simulink model "PlantaV4_6_prueba_contacto_4"  (R2021a)
settings: Solver=VariableStepAuto  StartTime=0.0  StopTime=60  MaxStep=1e-2  RelTol=1e-3
values from neighbouring files (symbols this model uses):
  ahmax = 0.75    [valoresPlanta_29_9_24.m]    (also in valoresPlanta_V3.m)
  alfahmax = ((2*ahmax)/(rhd))    (= 2)    [valoresPlanta_29_9_24.m]    (also in valoresPlanta_V3.m)
  alfatmax = atmax/rtd    (= 1.6)    [valoresPlanta_29_9_24.m]    (also in valoresPlanta_V3.m)
  atmax = 0.8    [valoresPlanta_29_9_24.m]    (also in valoresPlanta_V3.m)
  ax_max = 0.8    [valoresPlanta_29_9_24.m]    (also in valoresPlanta_v4.m)
  ay_max = 0.75    [valoresPlanta_29_9_24.m]    (also in valoresPlanta_v4.m)
  bcx = 1e6    (= 1000000)    [Valores_1.m]    (also in valoresPlanta.m; valoresPlanta_29_9_24.m; valoresPlanta_V3.m; valoresPlanta_v4.m)
  bcy = 1e7    (= 10000000)    [Valores_1.m]    (also in valoresPlanta.m; valoresPlanta_29_9_24.m; valoresPlanta_V3.m; valoresPlanta_v4.m)
  bh_eq = bhm*ih^2+bhd    (= 8720)    [Valores.m]    (also in Valores_1.m; valoresPlanta.m; valoresPlanta_29_9_24.m; valoresPlanta_V3.m)
  bhb = 1e8    (= 100000000)    [Valores.m]    (also in Valores_1.m; valoresPlanta.m; valoresPlanta_29_9_24.m; valoresPlanta_V3.m)
  bhEb = 2.2e9    (= 2200000000)    [Valores.m]    (also in Valores_1.m; valoresPlanta.m; valoresPlanta_29_9_24.m; valoresPlanta_V3.m)
  bt = 90.0    (= 90)    [Valores.m]    (also in Valores_1.m; valoresPlanta.m; valoresPlanta_29_9_24.m; valoresPlanta_V3.m)
  bt_eq = btd+(btm*(it^2))    (= 5401.8)    [valoresPlanta.m]    (also in valoresPlanta_29_9_24.m; valoresPlanta_V3.m; valoresPlanta_v4.m)
  btw = 3.0e3    (= 3000)    [Valores.m]    (also in Valores_1.m; valoresPlanta.m; valoresPlanta_29_9_24.m; valoresPlanta_V3.m)
  bwu = 150    [Valores.m]    (also in Valores_1.m; valoresPlanta.m; valoresPlanta_29_9_24.m; valoresPlanta_V3.m)
  estado_cont = [x_positions; hy_cont]    [perfilObsaculos.m]    (also in valoresPlanta_29_9_24.m = [x_positions; [hy_muelle hy_cont]])
  g = 9.80665    [Valores.m]    (also in Valores_1.m; valoresPlanta.m; valoresPlanta_29_9_24.m; valoresPlanta_V3.m)
  Hc = 0    [Valores.m]    (also in Valores_1.m = 2.5; valoresPlanta.m = 2.5; valoresPlanta_29_9_24.m = 2.5; valoresPlanta_V3.m = 2.5)
  hMax = 10    [Valores_1.m]    (also in valoresPlanta.m; valoresPlanta_V3.m; valoresPlanta_v4.m)
  hx_cont = 2.5    [perfilObsaculos.m]    (also in puntosTrayectoria.m; valoresPlanta_29_9_24.m)
  ih = 22    [Valores.m]    (also in Valores_1.m; valoresPlanta.m; valoresPlanta_29_9_24.m; valoresPlanta_V3.m)
  it = 30    [Valores.m]    (also in Valores_1.m; valoresPlanta.m; valoresPlanta_29_9_24.m; valoresPlanta_V3.m)
  Jh_eq = Jhm_hb*ih^2+Jhd_hEb    (= 18320)    [Valores.m]    (also in Valores_1.m; valoresPlanta.m; valoresPlanta_29_9_24.m; valoresPlanta_V3.m)
  Jt_eq = Jtd+(Jtm_tb*(it^2))    (= 7500)    [valoresPlanta.m]    (also in valoresPlanta_29_9_24.m; valoresPlanta_V3.m; valoresPlanta_v4.m)
  kcy = 1.8e9    (= 1800000000)    [Valores_1.m]    (also in valoresPlanta.m; valoresPlanta_29_9_24.m; valoresPlanta_V3.m; valoresPlanta_v4.m)
  KDh = Jeq2 * w_posh^3    (= -12245.4404091)    [Valores.m]    (also in Valores_1.m = Jeq2 * w_posh; valoresPlanta.m = Jeq2 * w_posh; valoresPlanta_29_9_24.m = Jh_eq * n * w_posh; valoresPlanta_V3.m = Jeq2 * w_posh)
  KDt = Meq2 * w_post^3    (= -4728.86946035)    [Valores.m]    (also in Valores_1.m = Meq2 * w_post; valoresPlanta.m = Meq2 * w_post; valoresPlanta_29_9_24.m = 10127; valoresPlanta_V3.m = Meq2 * w_post)
  KIh = Jeq2 * w_posh^2    (= 2572.66592082)    [Valores.m]    (also in Valores_1.m = Jeq2 * w_posh^3; valoresPlanta.m = Jeq2 * w_posh^3; valoresPlanta_29_9_24.m = Jh_eq * w_posh^3; valoresPlanta_V3.m = Jeq2 * w_posh^3)
  KIt = Meq2 * w_post^2    (= 1307.690244)    [Valores.m]    (also in Valores_1.m = Meq2 * w_post^3; valoresPlanta.m = Meq2 * w_post^3; valoresPlanta_29_9_24.m = 6809.6; valoresPlanta_V3.m = Meq2 * w_post^3)
  KPh = Jeq2 * w_posh    (= -540.495867769)    [Valores.m]    (also in Valores_1.m = Jeq2 * w_posh^2; valoresPlanta.m = Jeq2 * w_posh^2; valoresPlanta_29_9_24.m = Jh_eq * n * w_posh^2; valoresPlanta_V3.m = Jeq2 * w_posh^2)
  KPt = Meq2 * w_post    (= -361.62)    [Valores.m]    (also in Valores_1.m = Meq2 * w_post^2; valoresPlanta.m = Meq2 * w_post^2; valoresPlanta_29_9_24.m = 14123; valoresPlanta_V3.m = Meq2 * w_post^2)
  Ktw = 4.8e5    (= 480000)    [Valores.m]    (also in Valores_1.m; valoresPlanta.m; valoresPlanta_29_9_24.m; valoresPlanta_V3.m)
  kwu = 2.36e8    (= 236000000)    [Valores.m]    (also in Valores_1.m; valoresPlanta.m; valoresPlanta_29_9_24.m; valoresPlanta_V3.m)
  Mc_max = 5e4    (= 50000)    [Valores.m]    (also in Valores_1.m; valoresPlanta.m; valoresPlanta_29_9_24.m; valoresPlanta_V3.m)
  Mc_min = 2e3    (= 2000)    [Valores.m]    (also in Valores_1.m; valoresPlanta.m; valoresPlanta_29_9_24.m; valoresPlanta_V3.m)
  Meq = Mt+(it^2*Jtm_tb+Jtd)/rtd^2    (= 60000)    [Valores.m]    (also in Valores_1.m; valoresPlanta_29_9_24.m; valoresPlanta_v4.m)
  Ms = 1.5e4    (= 15000)    [Valores.m]    (also in Valores_1.m; valoresPlanta.m; valoresPlanta_29_9_24.m; valoresPlanta_V3.m)
  Mt = 30000    [Valores.m]    (also in Valores_1.m; valoresPlanta.m; valoresPlanta_29_9_24.m; valoresPlanta_V3.m)
  rhd = 0.75    [Valores.m]    (also in Valores_1.m; valoresPlanta.m; valoresPlanta_29_9_24.m; valoresPlanta_V3.m)
  rtd = 0.5    [Valores.m]    (also in Valores_1.m; valoresPlanta.m; valoresPlanta_29_9_24.m; valoresPlanta_V3.m)
  tau_hm = 1e-3    (= 0.001)    [valoresPlanta.m]    (also in valoresPlanta_29_9_24.m; valoresPlanta_V3.m; valoresPlanta_v4.m)
  tau_tm = 1e-3    (= 0.001)    [Valores.m]    (also in Valores_1.m; valoresPlanta.m; valoresPlanta_29_9_24.m; valoresPlanta_V3.m)
  Thb_Max = 5e4    (= 50000)    [Valores.m]    (also in Valores_1.m; valoresPlanta.m; valoresPlanta_29_9_24.m; valoresPlanta_V3.m)
  ThEb_Max = 1.1e6    (= 1100000)    [Valores.m]    (also in Valores_1.m; valoresPlanta.m; valoresPlanta_29_9_24.m; valoresPlanta_V3.m)
  Thm_Max = 2e4    (= 20000)    [Valores.m]    (also in Valores_1.m; valoresPlanta.m; valoresPlanta_29_9_24.m; valoresPlanta_V3.m)
  Ttb_Max = 5e3    (= 5000)    [Valores.m]    (also in Valores_1.m; valoresPlanta.m; valoresPlanta_29_9_24.m; valoresPlanta_V3.m)
  Ttm_Max = 3e3    (= 3000)    [Valores.m]    (also in Valores_1.m; valoresPlanta.m; valoresPlanta_29_9_24.m = 4000; valoresPlanta_V3.m)
  v_x_max = 4    [Valores_1.m]    (also in valoresPlanta.m; valoresPlanta_V3.m = 0.4; valoresPlanta_v4.m)
  vx_max = 4    [valoresPlanta_29_9_24.m]
  y0 = 2.5    [valoresPlanta_29_9_24.m]
  Yt0 = 45    [Valores.m]    (also in Valores_1.m; valoresPlanta.m; valoresPlanta_29_9_24.m; valoresPlanta_V3.m)
undefined symbols (not defined in the file or in its folder): sigbuilder_block, x0
libraries: vrlib x1, simulink_extras x1, cstblocks x1
(part 1 of 2)
settings Model: Creator=Matias  LastModifiedBy=agustin

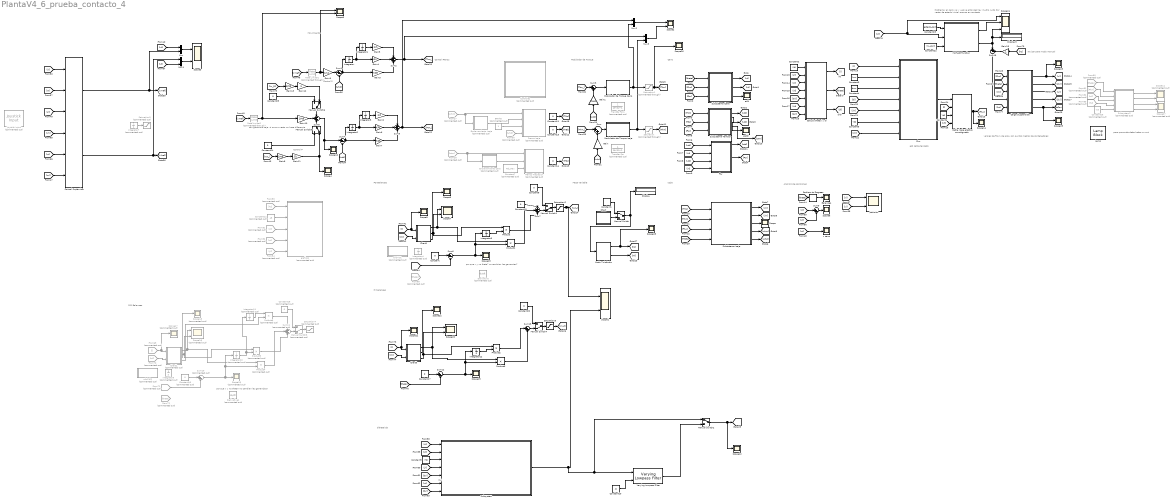
== system PlantaV4_6_prueba_contacto_4 ==
  note: para que ande debe haber un out
  note: revisar para modo manual
  note: ec2 cable tensado
  note: Problema: el carro va y vuelve entonces hay mucho ruido
      | Por vector de estado inicial arranco en contacto
  note: PI balanceo
  note: con ganancia baja, si sumo o resto no hace diferencia
  note: Control P
  note: por que v y no theta? no cambian las ganancias?
  note: d(theta)/dt
  note: Analisis de posiciones
  note: PD Balanceo
  note: Masa Variable
  note: Control Frenos
  note: Izaje
  note: Modulador de Torque
  note: Carro
  note: Movimiento
  note: PID Balanceo
  note: por que v y no theta? no cambian las ganancias?
  note: Control P
  note: valores de fila 1 de array son puntos medios de contenedores
  In4 : Inport
  BRKhE : Constant  Commented=on
  Balanceo : Scope
  Cable izaje elástico amortiguado : Subsystem
  Calculo theta,l y dl : Subsystem
  Carga Suspendida : Subsystem
  Chart : Stateflow chart  TreatAsAtomicUnit=on
  Chart1 : Stateflow chart  TreatAsAtomicUnit=on
  Chart2 : Stateflow chart  Commented=on  TreatAsAtomicUnit=on
  Chart3 : Stateflow chart  TreatAsAtomicUnit=on
  Constant{,8,11,13..15,17,20,24..25} (10 alike) : Constant  Value=0
  Constant1 : Constant  Value=65000
  Constant10 : Constant  Value=.8
  Constant12 : Constant  Commented=on  Value=45
  Constant16 : Constant  Commented=on  Value=0
  Constant18 : Constant  Commented=on  Value=0
  Constant{2,5..6,9} (4 alike) : Constant  Value=Yt0
  Constant22 : Constant  Value=hx_cont
  Constant23 : Constant  Value=estado_cont
  Constant26 : Constant  Commented=on  Value=-10
  Constant3 : Constant  Value=kwu
  Constant4 : Constant  Value=bwu
  Constant7 : Constant  Commented=on  Value=Ttb_Max
  Control Supervisor : Subsystem
  Controles : Subsystem  Commented=on
  Derivative : Derivative  Commented=on
  Derivative1 : Derivative  Commented=on
  Display : Display
  Display3 : Display
  Enclavamiento carro : Stateflow chart  Commented=on  TreatAsAtomicUnit=on
  Enclavamiento izaje : Stateflow chart  Commented=on  TreatAsAtomicUnit=on
  Fhw : Subsystem
  "Frenos Izaje " : Stateflow chart  Commented=on  TreatAsAtomicUnit=on
  Frenos Traslación : Stateflow chart  Commented=on  TreatAsAtomicUnit=on
  From27 : From  Commented=on  GotoTag=whm
  From28 : From  Commented=on  GotoTag=wtm
  From30 : From  Commented=on  GotoTag=whd
  From51 : From  Commented=on  GotoTag=xl
  From52 : From  Commented=on  GotoTag=xt
  From53 : From  Commented=on  GotoTag=hc
  From54 : From  Commented=on  GotoTag=yl
  From68 : From  Commented=on  GotoTag=theta
  From69 : From  Commented=on  GotoTag=l
  From70 : From  Commented=on  GotoTag=ml
  From71 : From  Commented=on  GotoTag=dTheta
  From72 : From  Commented=on  GotoTag=theta
  From80 : From  Commented=on  GotoTag=theta
  From81 : From  Commented=on  GotoTag=Fhw
  From82 : From  Commented=on  GotoTag=ml
  From83 : From  Commented=on  GotoTag=hc
  Ftw : Subsystem
  Gain : Gain  Gain=bh_eq
  Gain1 : Gain  Gain=bt_eq
  Gain10 : Gain  Gain=1/rtd
  Gain11 : Gain  Gain=.01
  Gain12 : Gain  Gain=.1
  Gain13 : Gain  Gain=1/rtd
  Gain15 : Gain
  Gain2 : Gain  Gain=KIt
  Gain3 : Gain  Gain=KDh
  Gain4 : Gain  Gain=KPh
  Gain5 : Gain  Gain=KIh
  Gain6 : Gain  Gain=KPt
  Gain7 : Gain  Gain=KDt
  Gain8 : Gain  Gain=1/rtd
  Gain9 : Gain  Gain=2/rhd
  Integrator{,1..3,5,12} (6 alike) : Integrator
  Integrator{4,7,9..11} (5 alike) : Integrator  Commented=on
  Joystick Input : vrlib/Joystick Input  Commented=on  joyid=1  adjustports=on  forcefeed=off
  Lamp : LampBlock
  MATLAB Function : MATLAB Function  TreatAsAtomicUnit=on
  Manual Switch : ManualSwitch
  Manual Switch{1,4..6} (4 alike) : ManualSwitch  CurrentSetting=0
  Manual Switch2 : ManualSwitch
  Manual Switch3 : ManualSwitch  Commented=on  CurrentSetting=0
  Modo Twistlocks : Stateflow chart  TreatAsAtomicUnit=on
  Modulador de Torque Carro : Subsystem
  Modulador de Torque Izaje : Subsystem
  Mux{,1..3} (4 alike) : Mux  Inputs=2
  Product{,1..2,6} (4 alike) : Product
  Product3 : Product  Commented=on
  Product4 : Product  Commented=on
  Product5 : Product  Commented=on
  Radians to Degrees : simulink_extras/Transformations/Radians to Degrees
  Rate Limiter1 : RateLimiter  Commented=through  RisingSlewLimit=ay_max  FallingSlewLimit=-ay_max  SampleTimeMode=inherited
  Rate Limiter2 : RateLimiter  Commented=through  RisingSlewLimit=ax_max  FallingSlewLimit=-ax_max  SampleTimeMode=inherited
  Saturation : Saturate  Commented=through  UpperLimit=Thm_Max  LowerLimit=-Thm_Max
  Saturation1 : Saturate  Commented=through  UpperLimit=Ttm_Max  LowerLimit=-Ttm_Max
  Saturation2 : Saturate  UpperLimit=4  LowerLimit=-4
  Saturation3 : Saturate  Commented=on  UpperLimit=v_x_max  LowerLimit=-4
  Saturation4 : Saturate  Commented=on  UpperLimit=4  LowerLimit=-4
  Saturation5 : Saturate  UpperLimit=4  LowerLimit=-4
  Scope{,4,6,8..10,12..14,19,21..23,25..26,28} (16 alike) : Scope
  Scope{1..3,5,7,20} (6 alike) : Scope  NumInputPorts=2
  Scope11 : Scope  Commented=on  NumInputPorts=2
  Scope15 : Scope  Commented=on
  Scope16 : Scope  Commented=on  NumInputPorts=2
  Scope17 : Scope  Commented=on
  Scope18 : Scope  Commented=on
  Scope24 : Scope  NumInputPorts=3
  Scope27 : Scope  Commented=on  NumInputPorts=2
  Subsistema Carro : Subsystem
  Subsistema Izaje : Subsystem
  Subsistema Tambor : Subsystem
  Subsystem : Subsystem
  Subsystem2 : Subsystem  Commented=on
  Sum : Sum  Inputs=|++
  Sum{1,4,6,9,12,15} (6 alike) : Sum  Inputs=|+-
  Sum10 : Sum  Commented=on  Inputs=|+-
  Sum11 : Sum  Commented=on  Inputs=+++
  Sum13 : Sum  Inputs=|++
  Sum2 : Sum  Inputs=+++
  Sum3 : Sum  Inputs=|++
  Sum5 : Sum  Inputs=+++
  Sum7 : Sum  Inputs=+++
  Sum8 : Sum  Inputs=-++
  Transfer Fcn : TransferFcn  Commented=on  Denominator=[1e-3 1]
  Transfer Fcn1 : TransferFcn  Commented=on  Denominator=[1e-3 1]
  Varying Lowpass Filter : cstblocks/Linear Parameter Varying/Varying Lowpass Filter  N=1
  at(t) : Scope
  atd(t) : Scope
  graficos : Stateflow chart  Commented=on  TreatAsAtomicUnit=on
  posicion : Scope  NumInputPorts=2
  whd*(t)1 : Subsystem  Tag=STV Subsys  Commented=on  LoadFcn=sigbuilder_block('load');  StartFcn=sigbuilder_block('start');  StopFcn=sigbuilder_block('stop');  ClipboardFcn=sigbuilder_block('clipboard');  mask(Sigbuilder block){tuvar=[0:10]}
      mask help: Simulink:masks:SigbuilderBlock_MD
      mask init:
      | if ~strcmp(get_param(bdroot(gcbh),'SimulationStatus'),'stopped') tuvar = sigbuilder_block('maskInit'); end
      settings: CopyFcn=sigbuilder_block('copy');  DeleteFcn=sigbuilder_block('delete');  ModelCloseFcn=sigbuilder_block('modelClose');  PreSaveFcn=sigbuilder_block('preSave');  PauseFcn=sigbuilder_block('pause');  ContinueFcn=sigbuilder_block('continue');  NameChangeFcn=sigbuilder_block('namechange');  OpenFcn=sigbuilder_block('open',[437.6 199.2 550.4 400 ]);  CloseFcn=sigbuilder_block('close');
      mask Display: plot(0, 0, 100, 100,[2, 2, 32, 32, 2], [68, 8, 8, 68, 68],[32, 2], [38, 38], [32, 19, 2],[53, 60, 44], [32, 17, 17, 2],[16, 16, 31, 31]);txt = getActiveGroup(gcbh);text(2, 100, txt,'verticalAlignment', 'top');
  whd*(t)2 : Subsystem  Tag=STV Subsys  Commented=on  LoadFcn=sigbuilder_block('load');  StartFcn=sigbuilder_block('start');  StopFcn=sigbuilder_block('stop');  ClipboardFcn=sigbuilder_block('clipboard');  mask(Sigbuilder block){tuvar=[0:10]}
      mask help: Simulink:masks:SigbuilderBlock_MD
      mask init:
      | if ~strcmp(get_param(bdroot(gcbh),'SimulationStatus'),'stopped') tuvar = sigbuilder_block('maskInit'); end
      settings: CopyFcn=sigbuilder_block('copy');  DeleteFcn=sigbuilder_block('delete');  ModelCloseFcn=sigbuilder_block('modelClose');  PreSaveFcn=sigbuilder_block('preSave');  PauseFcn=sigbuilder_block('pause');  ContinueFcn=sigbuilder_block('continue');  NameChangeFcn=sigbuilder_block('namechange');  OpenFcn=sigbuilder_block('open',[437.6 199.2 550.4 400 ]);  CloseFcn=sigbuilder_block('close');
      mask Display: plot(0, 0, 100, 100,[2, 2, 32, 32, 2], [68, 8, 8, 68, 68],[32, 2], [38, 38], [32, 19, 2],[53, 60, 44], [32, 17, 17, 2],[16, 16, 31, 31]);txt = getActiveGroup(gcbh);text(2, 100, txt,'verticalAlignment', 'top');
  x carro : Scope
  wires:
  Subsistema Tambor/1(xtd(t)) -> [xtd]
  Subsistema Tambor/2(vtd(t)) -> [vtd]
  Subsistema Carro/1(xt(t)) -> [xt]
  Subsistema Carro/2(vt(t)) -> [vt]
  Subsistema Carro/3(at(t)) -> at(t)/1
  Subsistema Tambor/3(atd(t)) -> atd(t)/1
  [Ttb] -> Subsistema Tambor/2(Ttb(t))
  [Ttm] -> Subsistema Tambor/1(Tm(t))
  [Ftw] -> Subsistema Carro/3(Ftw(t))
  [Fhw] -> Subsistema Carro/2(Fhw(t))
  [theta] -> Subsistema Carro/1(theta(t))
  [Ftw] -> Subsistema Tambor/3(Ftw(t))
  Ftw/1(Ftw(t)) -> [Ftw]
  [xtd] -> Ftw/1(xtd(t))
  [xt] -> Ftw/2(xt(t))
  [vtd] -> Ftw/3(vtd(t))
  [vt] -> Ftw/4(vt(t))
  [Thm] -> Subsistema Izaje/2(Thm(t))
  [Thb] -> Subsistema Izaje/1(Thb(t))
  [Fhw] -> Subsistema Izaje/3(Fhw(t))
  Subsistema Izaje/1(xh(t)) -> [xh]
  Subsistema Izaje/2(vh(t)) -> [vh]
  Subsistema Izaje/3(ah(t)) -> Scope/1
  Subsistema Izaje/4(whm(t)) -> [whm]
  Subsistema Tambor/4(wtm(t)) -> [wtm]
  [dxl] -> Calculo theta,l y dl/5(dxl)
  Constant2/1 -> Calculo theta,l y dl/1(Yt0)
  [yl] -> Calculo theta,l y dl/2(yl)
  Calculo theta,l y dl/3(dl) -> [dl]
  Calculo theta,l y dl/1(l) -> [l]
  [dyl] -> Calculo theta,l y dl/7(dyl)
  [xl] -> Calculo theta,l y dl/3(xl)
  [vt] -> Calculo theta,l y dl/6(vt)
  [xt] -> Calculo theta,l y dl/4(xt)
  Calculo theta,l y dl/2(theta) -> [theta]
  [dl] -> Fhw/4(dl(t))
  [xh] -> Fhw/7(xh(t))
  Constant3/1 -> Fhw/2(kwu)
  [l] -> Fhw/1(l(t))
  Constant5/1 -> Fhw/6(Yt0)
  [vh] -> Fhw/5(vh(t))
  Constant4/1 -> Fhw/3(bwu)
  Fhw/1(Fhw(t)) -> Cable izaje elástico amortiguado/1(Fhw)
  [l] -> Cable izaje elástico amortiguado/2(l(t))
  Constant6/1 -> Cable izaje elástico amortiguado/3(Yt0)
  [xh] -> Cable izaje elástico amortiguado/4(xh(t))
  Cable izaje elástico amortiguado/1(Fhw(t)) -> Scope14/1, [Fhw]
  [theta] -> Carga Suspendida/2(theta(t))
  [Fhw] -> Carga Suspendida/1(Fhw(t))
  Carga Suspendida/1(xl(t)) -> Scope23/1, [xl]
  Carga Suspendida/4(dyl(t)) -> [dyl]
  Carga Suspendida/3(yl(t)) -> [yl]
  Carga Suspendida/2(dxl(t)) -> [dxl]
  From27/1 -> "Frenos Izaje "/1(whm), Enclavamiento izaje/1(whm)
  From28/1 -> Enclavamiento carro/1(wtm), Frenos Traslación/1(wtm)
  Enclavamiento carro/1(BRKt) -> Frenos Traslación/2(BRKt)
  Enclavamiento izaje/1(BRKh) -> "Frenos Izaje "/2(BRKh)
  Constant7/1 -> Frenos Traslación/3(Ttb_Max)
  BRKhE/1 -> "Frenos Izaje "/3(BRKhE)
  Subsistema Izaje/5(whd(t)) -> [whd]
  [ThEb] -> Subsistema Izaje/4(ThEb(t))
  From30/1 -> "Frenos Izaje "/4(whd)
  [Thm_] -> Sum/1
  Sum/1 -> Modulador de Torque Izaje/1(Thm*(t))
  [whd] -> Gain/1
  Gain/1 -> Sum/2
  Integrator1/1 -> Gain5/1
  Integrator/1 -> Integrator1/1, Gain4/1
  Sum1/1 -> Integrator/1, Gain3/1
  Gain4/1 -> Sum2/2
  Gain5/1 -> Sum2/1
  Gain3/1 -> Sum2/3
  Sum3/1 -> Modulador de Torque Carro/1(Ttm*(t))
  [Ttm_] -> Sum3/1
  Gain1/1 -> Sum3/2
  Subsistema Tambor/5(wtd(t)) -> [wtd]
  [wtd] -> Gain1/1
  Gain7/1 -> Sum5/3
  [wtd] -> Sum4/2
  Gain6/1 -> Sum5/2
  Gain2/1 -> Sum5/1
  Integrator2/1 -> Integrator3/1, Gain6/1
  Sum4/1 -> Gain7/1, Integrator2/1
  Integrator3/1 -> Gain2/1
  [xl] -> posicion/1  "xl"
  [yl] -> posicion/2  "yl"
  [whd] -> Sum1/2
  Manual Switch/1 -> Modo Twistlocks/1(Mcx), Display/1
  [ml] -> Carga Suspendida/3(ml)
  [l] -> Scope8/1, Chart1/1(l)
  [ml] -> Chart1/2(ml)
  Product/1 -> Sum7/3
  Product1/1 -> Sum7/2
  Chart1/1(KD) -> Scope7/1, Product1/1
  Chart1/2(KP) -> Scope7/2, Product/1
  Constant/1 -> Sum6/1
  Sum8/1 -> Scope10/1, Sum4/1
  Sum7/1 -> Manual Switch1/2
  Chart/1(Mcx) -> Manual Switch/2
  Constant1/1 -> Manual Switch/1
  Constant8/1 -> Manual Switch1/1
  [yl] -> Control Supervisor/3(yl)
  Control Supervisor/2(vXref) -> Mux1/1, [vXref]  "vXref"
  Control Supervisor/1(vYref) -> Mux/2, [vYref]  "vYref"
  [xl] -> Control Supervisor/1(xl)
  Gain9/1 -> Sum1/1
  [ml] -> Control Supervisor/6(ml)
  Constant12/1 -> graficos/2(Yt0)
  From52/1 -> graficos/4(xt)
  From51/1 -> graficos/3(xl)
  From53/1 -> graficos/1(Hc)
  From54/1 -> graficos/5(yl)
  [xl] -> Sum9/1
  [xt] -> Sum9/2
  Sum9/1 -> Scope6/1
  [xt] -> x carro/1
  Radians to Degrees/1 -> Balanceo/1
  [theta] -> Radians to Degrees/1
  Chart1/3(WN) -> Scope9/1
  Integrator5/1 -> Product/2
  Gain8/1 -> Gain11/1
  Gain11/1 -> Scope4/1, Manual Switch5/2
  [Vxt_] -> Gain8/1
  Gain10/1 -> Sum8/2
  [xt] -> Control Supervisor/2(xt)
  [dyl] -> Subsystem/7(d(yl(t))/dt)
  [vt] -> Subsystem/6(d(xt(t))/dt)
  [dxl] -> Subsystem/5(d(xl(t))/dt)
  [yl] -> Subsystem/4(yl(t))
  [xt] -> Subsystem/2(xt(t))
  [xl] -> Subsystem/1(xl(t))
  Constant9/1 -> Subsystem/3(Yto)
  [vXref] -> Rate Limiter2/1  "vXref"
  [vYref] -> Rate Limiter1/1  "vYref"
  Sum2/1 -> [Thm_], Mux3/1  "Thm_"
  Sum5/1 -> [Ttm_], Mux2/1  "Ttm_"
  Manual Switch1/1 -> Saturation2/1
  [dTheta] -> Sum6/2
  Saturation2/1 -> Scope1/1, [Vxt_]
  Rate Limiter1/1 -> Scope5/1, Gain9/1
  Rate Limiter2/1 -> Gain10/1, Scope5/2
  [vh] -> Control Supervisor/4(vh)
  [vt] -> Control Supervisor/5(vt)
  [vh] -> Mux/1
  [vt] -> Mux1/2
  Mux1/1 -> Scope3/2
  Mux/1 -> Scope3/1
  Subsystem/1(d(theta(t))/dt) -> Manual Switch2/1, Varying Lowpass Filter/1, Scope1/2
  Varying Lowpass Filter/1 -> Manual Switch2/2
  Constant10/1 -> Varying Lowpass Filter/2
  Manual Switch2/1 -> Scope12/1, [dTheta]
  Sum6/1 -> Scope13/1, Product1/2, Integrator5/1
  Mux2/1 -> Scope2/1
  Mux3/1 -> Scope2/2
  Constant11/1 -> [Thb]
  Constant13/1 -> [ThEb]
  Constant14/1 -> [Ttb]
  Integrator7/1 -> Saturation3/1  "vXref"
  Constant15/1 -> Sum7/1
  Chart2/4(KI) -> Product5/2
  Product3/1 -> Sum11/3
  Sum11/1 -> Manual Switch3/2
  Chart2/2(KP) -> Product3/1, Scope16/2
  Integrator11/1 -> Product5/1
  From71/1 -> Sum10/2
  Integrator10/1 -> Integrator11/1, Product3/2
  Chart2/3(WN) -> Scope18/1
  Constant18/1 -> Manual Switch3/1
  Constant16/1 -> Sum10/1
  Chart2/1(KD) -> Scope16/1, Product4/1
  From70/1 -> Chart2/2(ml)
  Product4/1 -> Sum11/2
  From69/1 -> Scope17/1, Chart2/1(l)
  Sum10/1 -> Scope15/1, Product4/2, Integrator10/1
  Manual Switch3/1 -> Saturation4/1
  Product5/1 -> Sum11/1
  [theta] -> Sum12/2
  Chart3/3(KI) -> Scope20/2, Product2/1
  [ml] -> Chart3/2(ml)
  [l] -> Scope21/1, Chart3/1(l)
  Manual Switch4/1 -> Saturation5/1
  Integrator12/1 -> Product2/2
  Chart3/2(WN) -> Scope22/1
  Sum12/1 -> Scope19/1, Product6/2, Integrator12/1
  Chart3/1(KP) -> Product6/1, Scope20/1
  Product6/1 -> Sum13/2
  Sum13/1 -> Manual Switch4/2
  Constant20/1 -> Manual Switch4/1
  Product2/1 -> Sum13/1
  Constant17/1 -> Sum12/1
  Saturation5/1 -> [Vx_PI]
  Manual Switch6/1 -> Sum8/1
  Gain13/1 -> Gain12/1
  [Vx_PI] -> Gain13/1
  Modo Twistlocks/1(hc) -> Scope28/1, [hc]
  Modo Twistlocks/2(ml) -> [ml]
  [hc] -> Carga Suspendida/5(hc)
  Constant22/1 -> MATLAB Function/3(anchoCont)
  Constant23/1 -> MATLAB Function/1(estado_cont)
  [xt] -> Scope24/1, MATLAB Function/2(xl)
  Gain15/1 -> Sum15/2
  [hc] -> Gain15/1
  MATLAB Function/1(index) -> Scope24/2
  Constant24/1 -> Manual Switch5/1
  Manual Switch5/1 -> Sum8/3
  Gain12/1 -> Manual Switch6/2
  Constant25/1 -> Manual Switch6/1
  Modulador de Torque Carro/1(Ttm(t)) -> Saturation1/1, Mux2/2
  Modulador de Torque Izaje/1(Thm(t)) -> Saturation/1, Mux3/2
  Saturation1/1 -> Scope26/1, [Ttm]
  Saturation/1 -> [Thm]
  From80/1 -> Subsystem2/1(Theta)
  From81/1 -> Subsystem2/2(Fhw1)
  From82/1 -> Subsystem2/3(ml)
  From83/1 -> Subsystem2/4(hc)
  Subsystem2/1(xl) -> Scope11/1
  Subsystem2/2(yl) -> Scope11/2
  Subsystem2/3(xl') -> Scope27/1
  Subsystem2/4(yl') -> Scope27/2
  MATLAB Function/2(y_evol) -> Display3/1, Scope24/3, Sum15/1
  Constant26/1 -> Subsystem2/5(yc0)
  Sum15/1 -> Carga Suspendida/4(yc0)
  Carga Suspendida/5(estadoContacto) -> Scope25/1, [eCon]

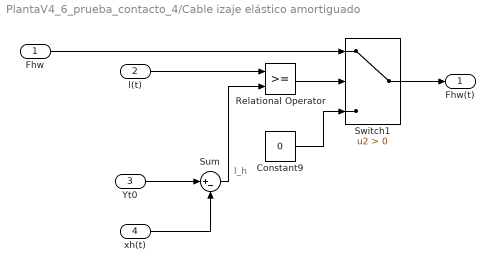
== system PlantaV4_6_prueba_contacto_4/Cable izaje elástico amortiguado ==
  note: l_h
  Fhw : Inport
  l(t) : Inport  Port=2
  Yt0 : Inport  Port=3
  xh(t) : Inport  Port=4
  Constant9 : Constant  Value=0
  Relational Operator : RelationalOperator  OutDataTypeStr=boolean  RndMeth=Simplest
  Sum : Sum  Inputs=|+-
  Switch1 : Switch  Criteria=u2 > Threshold
  Fhw(t) : Outport
  wires:
  l(t)/1 -> Relational Operator/1
  Sum/1 -> Relational Operator/2
  Fhw/1 -> Switch1/1
  Yt0/1 -> Sum/1
  Constant9/1 -> Switch1/3
  Relational Operator/1 -> Switch1/2
  xh(t)/1 -> Sum/2
  Switch1/1 -> Fhw(t)/1

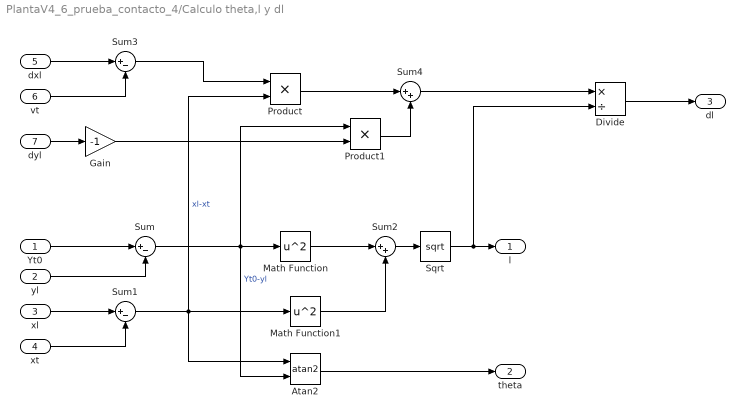
== system PlantaV4_6_prueba_contacto_4/Calculo theta,l y dl ==
  Yt0 : Inport
  yl : Inport  Port=2
  xl : Inport  Port=3
  xt : Inport  Port=4
  dxl : Inport  Port=5
  vt : Inport  Port=6
  dyl : Inport  Port=7
  Atan2 : Trigonometry  Operator=atan2
  Divide : Product  Inputs=*/
  Gain : Gain  Gain=-1
  Math Function : Math  Operator=square  SaturateOnIntegerOverflow=on
  Math Function1 : Math  Operator=square  SaturateOnIntegerOverflow=on
  Product : Product
  Product1 : Product
  Sqrt : Sqrt  SaturateOnIntegerOverflow=on
  Sum : Sum  Inputs=|+-
  Sum1 : Sum  Inputs=|+-
  Sum2 : Sum  Inputs=|++
  Sum3 : Sum  Inputs=|+-
  Sum4 : Sum  Inputs=|++
  l : Outport
  theta : Outport  Port=2
  dl : Outport  Port=3
  wires:
  Yt0/1 -> Sum/1
  yl/1 -> Sum/2
  xl/1 -> Sum1/1
  xt/1 -> Sum1/2
  Atan2/1 -> theta/1
  Sum1/1 -> Product/2, Math Function1/1, Atan2/1  "xl-xt"
  Sum/1 -> Product1/1, Atan2/2, Math Function/1  "Yt0-yl"
  Math Function/1 -> Sum2/1
  Math Function1/1 -> Sum2/2
  Sum2/1 -> Sqrt/1
  Sqrt/1 -> Divide/2, l/1
  dxl/1 -> Sum3/1
  vt/1 -> Sum3/2
  Sum3/1 -> Product/1
  dyl/1 -> Gain/1
  Gain/1 -> Product1/2
  Product/1 -> Sum4/1
  Product1/1 -> Sum4/2
  Sum4/1 -> Divide/1
  Divide/1 -> dl/1

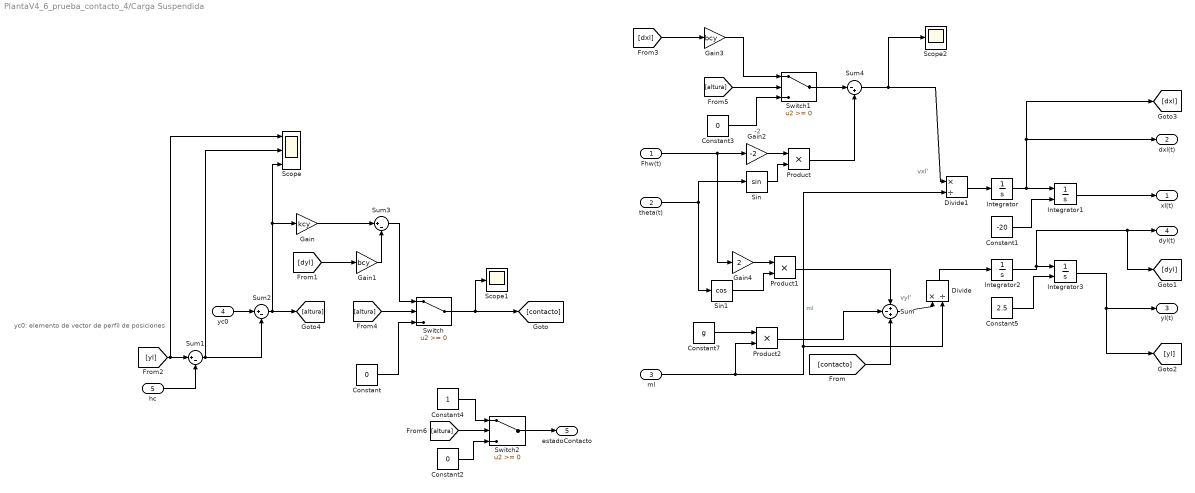
== system PlantaV4_6_prueba_contacto_4/Carga Suspendida ==
  note: -2
  note: vxl'
  note: vyl'
  note: yc0: elemento de vector de perfil de posiciones
  Fhw(t) : Inport
  theta(t) : Inport  Port=2
  ml : Inport  Port=3
  yc0 : Inport  Port=4
  hc : Inport  Port=5
  Constant : Constant  Value=0
  Constant1 : Constant  Value=-20
  Constant2 : Constant  Value=0
  Constant3 : Constant  Value=0
  Constant4 : Constant
  Constant5 : Constant  Value=2.5
  Constant7 : Constant  Value=g
  Divide : Product  Inputs=*/
  Divide1 : Product  Inputs=*/
  Gain : Gain  Gain=kcy
  Gain1 : Gain  Gain=bcy
  Gain2 : Gain  Gain=-2
  Gain3 : Gain  Gain=bcy
  Gain4 : Gain  Gain=2
  Integrator : Integrator
  Integrator1 : Integrator  InitialConditionSource=external
  Integrator2 : Integrator
  Integrator3 : Integrator  InitialConditionSource=external
  Product : Product
  Product1 : Product
  Product2 : Product
  Scope : Scope  NumInputPorts=3
  Scope1 : Scope
  Scope2 : Scope
  Sin : Trigonometry
  Sin1 : Trigonometry  Operator=cos
  Sum : Sum  Inputs=+-+
  Sum1 : Sum  Inputs=|+-
  Sum2 : Sum  Inputs=|+-
  Sum3 : Sum  Inputs=|+-
  Sum4 : Sum  Inputs=|-+
  Switch : Switch
  Switch1 : Switch
  Switch2 : Switch
  xl(t) : Outport
  dxl(t) : Outport  Port=2
  yl(t) : Outport  Port=3
  dyl(t) : Outport  Port=4
  estadoContacto : Outport  Port=5
  wires:
  Divide1/1 -> Integrator/1
  theta(t)/1 -> Sin1/1, Sin/1
  Constant7/1 -> Product2/1
  Product2/1 -> Sum/2
  Product/1 -> Sum4/2
  Fhw(t)/1 -> Gain4/1, Gain2/1
  Sum/1 -> Divide/1
  Integrator/1 -> [dxl], dxl(t)/1, Integrator1/1
  Sin1/1 -> Product1/2
  Gain2/1 -> Product/1
  Product1/1 -> Sum/1
  Sin/1 -> Product/2
  Integrator1/1 -> xl(t)/1
  Integrator2/1 -> [dyl], dyl(t)/1, Integrator3/1
  Divide/1 -> Integrator2/1
  Gain4/1 -> Product1/1
  Integrator3/1 -> [yl], yl(t)/1
  ml/1 -> Product2/2, Divide1/2, Divide/2  "ml"
  [yl] -> Scope/1, Sum1/1
  hc/1 -> Sum1/2
  Sum1/1 -> Scope/2, Sum2/2
  yc0/1 -> Sum2/1
  Constant/1 -> Switch/3
  [dyl] -> Gain1/1
  Gain1/1 -> Sum3/2
  Gain/1 -> Sum3/1
  Sum2/1 -> [altura], Scope/3, Gain/1
  Sum3/1 -> Switch/1
  Switch/1 -> Scope1/1, [contacto]
  [contacto] -> Sum/3
  Constant1/1 -> Integrator1/2
  [dxl] -> Gain3/1
  [altura] -> Switch/2
  [altura] -> Switch1/2
  Constant3/1 -> Switch1/3
  Gain3/1 -> Switch1/1
  Switch1/1 -> Sum4/1
  Sum4/1 -> Scope2/1, Divide1/1
  Switch2/1 -> estadoContacto/1
  Constant2/1 -> Switch2/3
  Constant4/1 -> Switch2/1
  [altura] -> Switch2/2
  Constant5/1 -> Integrator3/2

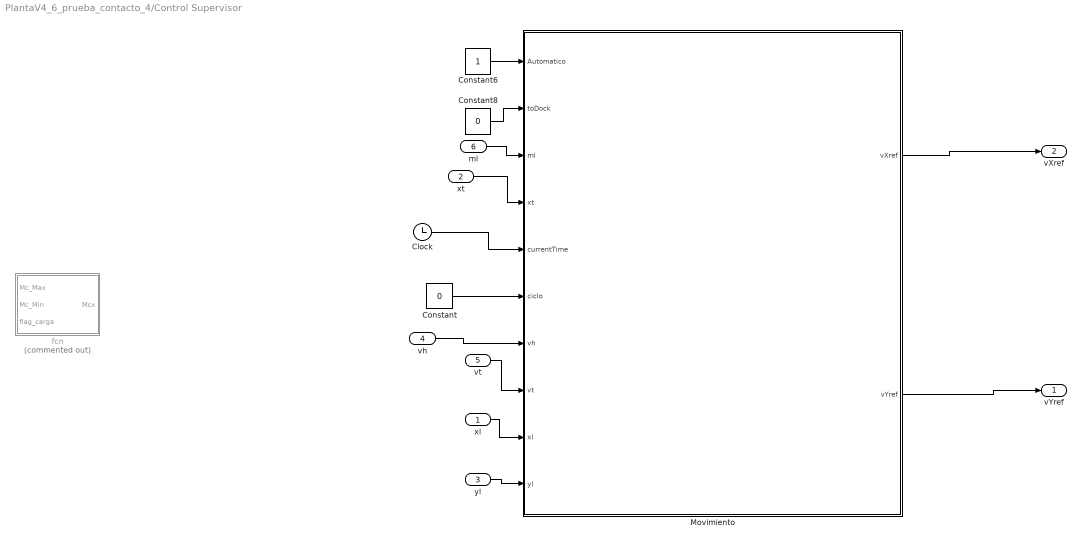
== system PlantaV4_6_prueba_contacto_4/Control Supervisor ==
  xl : Inport
  xt : Inport  Port=2
  yl : Inport  Port=3
  vh : Inport  Port=4
  vt : Inport  Port=5
  ml : Inport  Port=6
  Clock : Clock
  Constant : Constant  Value=0
  Constant6 : Constant
  Constant8 : Constant  Value=0
  Movimiento : Stateflow chart  TreatAsAtomicUnit=on
      settings: PortSchema="{\"entries\":[{\"content\":{\"sides\":[{\"content\":{\"connectorIds\":[\"In1\",\"In2\",\"In7\",\"In8\",\"In9\",\"In10\",\"In5\",\"In6\",\"In3\",\"In4\"]},\"type\":\"ConnectorPlacement.EquallySpacedRectSide\",\"uuid\":\"7754e6e1-1487-4c5e-b93c-5b95548dc503\"},{\"content\":{\"connectorIds\":[\"Out1\",\"Out2\"],\"side\":\"RIGHT\"},\"type\":\"ConnectorPlacement.EquallySpacedRectSide\",\"uuid\":\"e49bdf6e-b30d-4ce2-b56a-406d79434d70\"},{\"content\":{\"connectorIds\":[],\"side\":\"TOP\"},\"type\":\"ConnectorPlacement.EquallySpacedRectSide\",\"uuid\":\"816dde99-88b4-4e51-8e7c-8334ef27840c\"}]},\"type\":\"ConnectorPlacement.EquallySpacedConnector\",\"uuid\":\"e43ca6b0-ace3-4be2-8389-da1b8832a6a4\"}],\"packageUris\":[\"http://schema.mathworks.com/mf0/Connector/R2020b\"],\"version\":\"1.0\"}"
  fcn : MATLAB Function  Commented=on  TreatAsAtomicUnit=on
  vYref : Outport
  vXref : Outport  Port=2
  wires:
  Constant6/1 -> Movimiento/1(Automatico)
  Constant8/1 -> Movimiento/2(toDock)
  xl/1 -> Movimiento/3(xl)
  yl/1 -> Movimiento/4(yl)
  ml/1 -> Movimiento/7(ml)
  xt/1 -> Movimiento/8(xt)
  vh/1 -> Movimiento/5(vh)
  vt/1 -> Movimiento/6(vt)
  Clock/1 -> Movimiento/9(currentTime)
  Movimiento/1(vXref) -> vXref/1
  Movimiento/2(vYref) -> vYref/1
  Constant/1 -> Movimiento/10(ciclo)

== system PlantaV4_6_prueba_contacto_4/Controles ==
  Lamp : LampBlock
  Lamp1 : LampBlock
  Lamp2 : LampBlock
  Rocker Switch : RockerSwitchBlock
      settings: Values={{'Off', 'On'}, [0 1]}
  Rocker Switch1 : RockerSwitchBlock
      settings: Values={{'Off', 'On'}, [0 1]}
  Rocker Switch2 : RockerSwitchBlock
      settings: Values={{'Off', 'On'}, [0 1]}

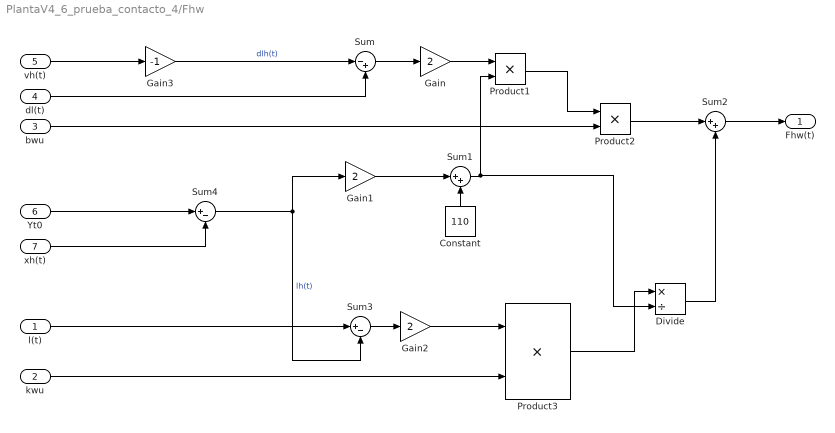
== system PlantaV4_6_prueba_contacto_4/Fhw ==
  l(t) : Inport
  kwu : Inport  Port=2
  bwu : Inport  Port=3
  dl(t) : Inport  Port=4
  vh(t) : Inport  Port=5
  Yt0 : Inport  Port=6
  xh(t) : Inport  Port=7
  Constant : Constant  Value=110
  Divide : Product  Inputs=*/
  Gain : Gain  Gain=2
  Gain1 : Gain  Gain=2
  Gain2 : Gain  Gain=2
  Gain3 : Gain  Gain=-1
  Product1 : Product
  Product2 : Product
  Product3 : Product
  Sum : Sum  Inputs=|-+
  Sum1 : Sum  Inputs=|++
  Sum2 : Sum  Inputs=|++
  Sum3 : Sum  Inputs=|+-
  Sum4 : Sum  Inputs=|+-
  Fhw(t) : Outport
  wires:
  dl(t)/1 -> Sum/2
  Sum/1 -> Gain/1
  Gain1/1 -> Sum1/1
  Sum4/1 -> Sum3/2, Gain1/1  "lh(t)"
  l(t)/1 -> Sum3/1
  Constant/1 -> Sum1/2
  Gain/1 -> Product1/1
  Sum1/1 -> Product1/2, Divide/2
  Product1/1 -> Product2/1
  bwu/1 -> Product2/2
  Product2/1 -> Sum2/1
  Sum3/1 -> Gain2/1
  Gain2/1 -> Product3/1
  kwu/1 -> Product3/2
  Product3/1 -> Divide/1
  Divide/1 -> Sum2/2
  Sum2/1 -> Fhw(t)/1
  vh(t)/1 -> Gain3/1
  Gain3/1 -> Sum/1  "dlh(t)"
  Yt0/1 -> Sum4/1
  xh(t)/1 -> Sum4/2

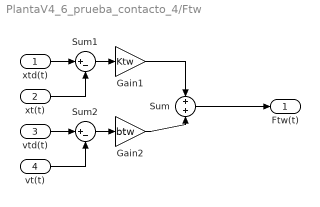
== system PlantaV4_6_prueba_contacto_4/Ftw ==
  xtd(t) : Inport
  xt(t) : Inport  Port=2
  vtd(t) : Inport  Port=3
  vt(t) : Inport  Port=4
  Gain1 : Gain  Gain=Ktw
  Gain2 : Gain  Gain=btw
  Sum : Sum
  Sum1 : Sum  Inputs=|+-
  Sum2 : Sum  Inputs=|+-
  Ftw(t) : Outport
  wires:
  Sum2/1 -> Gain2/1
  xtd(t)/1 -> Sum1/1
  vt(t)/1 -> Sum2/2
  xt(t)/1 -> Sum1/2
  Sum/1 -> Ftw(t)/1
  vtd(t)/1 -> Sum2/1
  Gain2/1 -> Sum/2
  Gain1/1 -> Sum/1
  Sum1/1 -> Gain1/1

== system PlantaV4_6_prueba_contacto_4/Modulador de Torque Carro ==
  Ttm*(t) : Inport
  Gain1 : Gain  Gain=1/tau_tm
  Integrator : Integrator
  Sum : Sum  Inputs=|+-
  Ttm(t) : Outport
  wires:
  Gain1/1 -> Integrator/1
  Integrator/1 -> Ttm(t)/1, Sum/2
  Ttm*(t)/1 -> Sum/1
  Sum/1 -> Gain1/1

== system PlantaV4_6_prueba_contacto_4/Modulador de Torque Izaje ==
  Thm*(t) : Inport
  Gain1 : Gain  Gain=1/tau_hm
  Integrator : Integrator
  Sum : Sum  Inputs=|+-
  Thm(t) : Outport
  wires:
  Gain1/1 -> Integrator/1
  Integrator/1 -> Thm(t)/1, Sum/2
  Thm*(t)/1 -> Sum/1
  Sum/1 -> Gain1/1

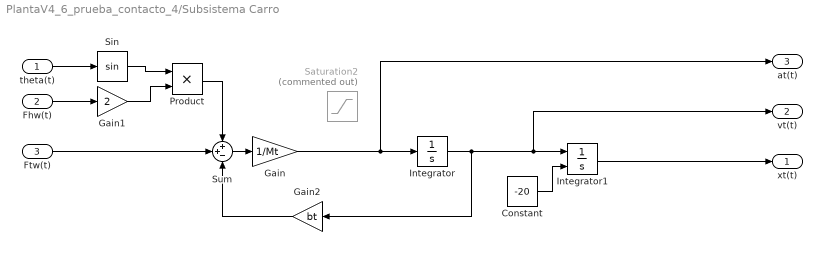
== system PlantaV4_6_prueba_contacto_4/Subsistema Carro ==
  theta(t) : Inport
  Fhw(t) : Inport  Port=2
  Ftw(t) : Inport  Port=3
  Constant : Constant  Value=-20
  Gain : Gain  Gain=1/Mt
  Gain1 : Gain  Gain=2
  Gain2 : Gain  Gain=bt
  Integrator : Integrator
  Integrator1 : Integrator  InitialConditionSource=external
  Product : Product
  Saturation2 : Saturate  Commented=on  UpperLimit=atmax  LowerLimit=-atmax
  Sin : Trigonometry
  Sum : Sum  Inputs=++-
  xt(t) : Outport
  vt(t) : Outport  Port=2
  at(t) : Outport  Port=3
  wires:
  Integrator/1 -> vt(t)/1, Integrator1/1, Gain2/1
  Gain1/1 -> Product/2
  theta(t)/1 -> Sin/1
  Sum/1 -> Gain/1
  Product/1 -> Sum/1
  Integrator1/1 -> xt(t)/1
  Ftw(t)/1 -> Sum/2
  Gain2/1 -> Sum/3
  Fhw(t)/1 -> Gain1/1
  Sin/1 -> Product/1
  Gain/1 -> at(t)/1, Integrator/1
  Constant/1 -> Integrator1/2

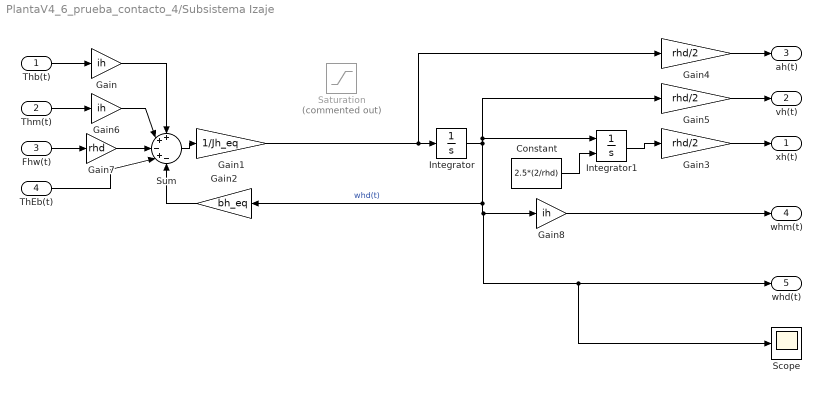
== system PlantaV4_6_prueba_contacto_4/Subsistema Izaje ==
  Thb(t) : Inport
  Thm(t) : Inport  Port=2
  Fhw(t) : Inport  Port=3
  ThEb(t) : Inport  Port=4
  Constant : Constant  Value=2.5*(2/rhd)
  Gain : Gain  Gain=ih
  Gain1 : Gain  Gain=1/Jh_eq
  Gain2 : Gain  Gain=bh_eq
  Gain3 : Gain  Gain=rhd/2
  Gain4 : Gain  Gain=rhd/2
  Gain5 : Gain  Gain=rhd/2
  Gain6 : Gain  Gain=ih
  Gain7 : Gain  Gain=rhd
  Gain8 : Gain  Gain=ih
  Integrator : Integrator
  Integrator1 : Integrator  InitialConditionSource=external
  Saturation : Saturate  Commented=on  UpperLimit=alfahmax  LowerLimit=-alfahmax
  Scope : Scope
  Sum : Sum  Inputs=++-+-
  xh(t) : Outport
  vh(t) : Outport  Port=2
  ah(t) : Outport  Port=3
  whm(t) : Outport  Port=4
  whd(t) : Outport  Port=5
  wires:
  Integrator/1 -> Gain5/1, Integrator1/1, Scope/1, whd(t)/1, Gain8/1, Gain2/1  "whd(t)"
  Gain2/1 -> Sum/5
  Gain4/1 -> ah(t)/1
  Gain3/1 -> xh(t)/1
  Gain5/1 -> vh(t)/1
  Fhw(t)/1 -> Gain7/1
  Integrator1/1 -> Gain3/1
  Thb(t)/1 -> Gain/1
  Gain1/1 -> Gain4/1, Integrator/1
  Sum/1 -> Gain1/1
  Thm(t)/1 -> Gain6/1
  Gain/1 -> Sum/1
  Gain6/1 -> Sum/2
  Gain7/1 -> Sum/3
  ThEb(t)/1 -> Sum/4
  Gain8/1 -> whm(t)/1
  Constant/1 -> Integrator1/2

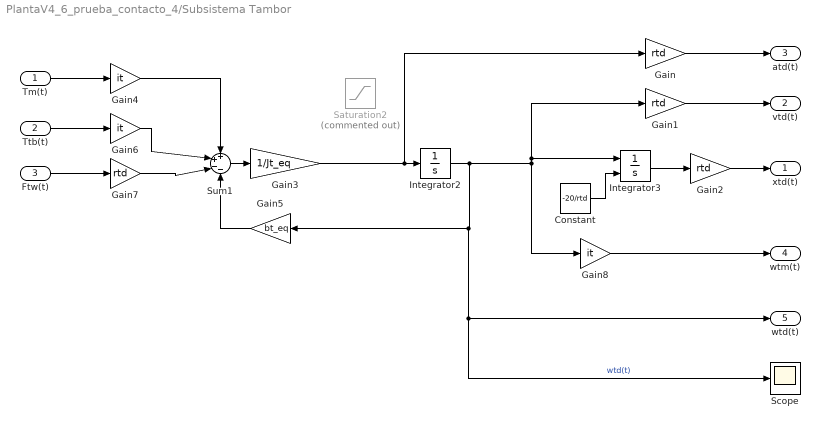
== system PlantaV4_6_prueba_contacto_4/Subsistema Tambor ==
  Tm(t) : Inport
  Ttb(t) : Inport  Port=2
  Ftw(t) : Inport  Port=3
  Constant : Constant  Value=-20/rtd
  Gain{,1..2,7} (4 alike) : Gain  Gain=rtd
  Gain3 : Gain  Gain=1/Jt_eq
  Gain4 : Gain  Gain=it
  Gain5 : Gain  Gain=bt_eq
  Gain6 : Gain  Gain=it
  Gain8 : Gain  Gain=it
  Integrator2 : Integrator
  Integrator3 : Integrator  InitialConditionSource=external
  Saturation2 : Saturate  Commented=on  UpperLimit=alfatmax  LowerLimit=-alfatmax
  Scope : Scope
  Sum1 : Sum  Inputs=++--
  xtd(t) : Outport
  vtd(t) : Outport  Port=2
  atd(t) : Outport  Port=3
  wtm(t) : Outport  Port=4
  wtd(t) : Outport  Port=5
  wires:
  Integrator3/1 -> Gain2/1
  Ftw(t)/1 -> Gain7/1
  Gain2/1 -> xtd(t)/1
  Integrator2/1 -> Gain1/1, Integrator3/1, Gain8/1, Scope/1, wtd(t)/1, Gain5/1  "wtd(t)"
  Tm(t)/1 -> Gain4/1
  Ttb(t)/1 -> Gain6/1
  Sum1/1 -> Gain3/1
  Gain5/1 -> Sum1/4
  Gain1/1 -> vtd(t)/1
  Gain/1 -> atd(t)/1
  Gain4/1 -> Sum1/1
  Gain6/1 -> Sum1/2
  Gain7/1 -> Sum1/3
  Gain8/1 -> wtm(t)/1
  Gain3/1 -> Gain/1, Integrator2/1
  Constant/1 -> Integrator3/2

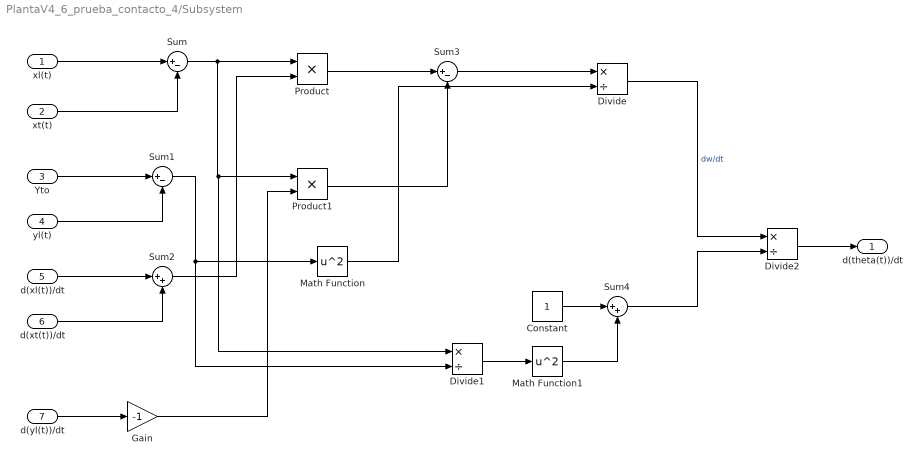
== system PlantaV4_6_prueba_contacto_4/Subsystem ==
  xl(t) : Inport
  xt(t) : Inport  Port=2
  Yto : Inport  Port=3
  yl(t) : Inport  Port=4
  d(xl(t))/dt : Inport  Port=5
  d(xt(t))/dt : Inport  Port=6
  d(yl(t))/dt : Inport  Port=7
  Constant : Constant
  Divide : Product  Inputs=*/
  Divide1 : Product  Inputs=*/
  Divide2 : Product  Inputs=*/
  Gain : Gain  Gain=-1
  Math Function : Math  Operator=square  SaturateOnIntegerOverflow=on
  Math Function1 : Math  Operator=square  SaturateOnIntegerOverflow=on
  Product : Product
  Product1 : Product
  Sum : Sum  Inputs=|+-
  Sum1 : Sum  Inputs=|+-
  Sum2 : Sum  Inputs=|++
  Sum3 : Sum  Inputs=|+-
  Sum4 : Sum  Inputs=|++
  d(theta(t))/dt : Outport
  wires:
  xl(t)/1 -> Sum/1
  xt(t)/1 -> Sum/2
  Yto/1 -> Sum1/1
  yl(t)/1 -> Sum1/2
  Sum/1 -> Divide1/1, Product1/1, Product/1
  d(xl(t))/dt/1 -> Sum2/1
  d(xt(t))/dt/1 -> Sum2/2
  Sum2/1 -> Product/2
  Product/1 -> Sum3/1
  Product1/1 -> Sum3/2
  d(yl(t))/dt/1 -> Gain/1
  Gain/1 -> Product1/2
  Sum3/1 -> Divide/1
  Sum1/1 -> Math Function/1, Divide1/2
  Math Function/1 -> Divide/2
  Divide/1 -> Divide2/1  "dw/dt"
  Divide1/1 -> Math Function1/1
  Math Function1/1 -> Sum4/2
  Constant/1 -> Sum4/1
  Divide2/1 -> d(theta(t))/dt/1
  Sum4/1 -> Divide2/2

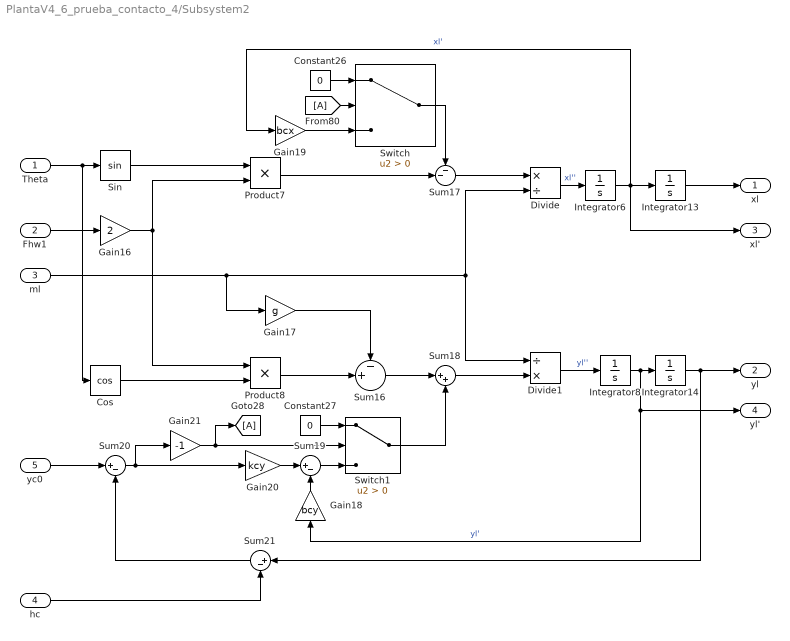
== system PlantaV4_6_prueba_contacto_4/Subsystem2 ==
  Theta : Inport
  Fhw1 : Inport  Port=2
  ml : Inport  Port=3
  hc : Inport  Port=4
  yc0 : Inport  Port=5
  Constant26 : Constant  Value=0
  Constant27 : Constant  Value=0
  Cos : Trigonometry  Operator=cos
  Divide : Product  Inputs=*/
  Divide1 : Product  Inputs=/*
  Gain16 : Gain  Gain=2
  Gain17 : Gain  Gain=g
  Gain18 : Gain  Gain=bcy
  Gain19 : Gain  Gain=bcx
  Gain20 : Gain  Gain=kcy
  Gain21 : Gain  Gain=-1
  Integrator13 : Integrator  InitialCondition=x0
  Integrator14 : Integrator  InitialCondition=y0
  Integrator6 : Integrator
  Integrator8 : Integrator
  Product7 : Product
  Product8 : Product
  Sin : Trigonometry
  Sum16 : Sum  Inputs=-+|
  Sum17 : Sum  Inputs=--|
  Sum18 : Sum  Inputs=|++
  Sum19 : Sum  Inputs=|+-
  Sum20 : Sum  Inputs=|+-
  Sum21 : Sum  Inputs=|+-
  Switch : Switch  Criteria=u2 > Threshold
  Switch1 : Switch  Criteria=u2 > Threshold
  xl : Outport
  yl : Outport  Port=2
  xl' : Outport  Port=3
  yl' : Outport  Port=4
  wires:
  Sum20/1 -> Gain21/1, Gain20/1
  Product7/1 -> Sum17/2
  Integrator13/1 -> xl/1
  Sum18/1 -> Divide1/2
  Integrator6/1 -> xl'/1, Gain19/1, Integrator13/1  "xl'"
  Gain19/1 -> Switch/3
  Gain20/1 -> Sum19/1
  Gain17/1 -> Sum16/1
  Integrator8/1 -> yl'/1, Gain18/1, Integrator14/1  "yl'"
  Gain16/1 -> Product8/1, Product7/2
  Divide/1 -> Integrator6/1  "xl''"
  Sum17/1 -> Divide/1
  yc0/1 -> Sum20/1
  Gain21/1 -> [A], Switch1/2
  Cos/1 -> Product8/2
  hc/1 -> Sum21/2
  Sum21/1 -> Sum20/2
  Constant27/1 -> Switch1/1
  Gain18/1 -> Sum19/2
  ml/1 -> Gain17/1, Divide/2, Divide1/1
  Integrator14/1 -> yl/1, Sum21/1
  Switch1/1 -> Sum18/2
  Theta/1 -> Cos/1, Sin/1
  Constant26/1 -> Switch/1
  [A] -> Switch/2
  Switch/1 -> Sum17/1
  Sum19/1 -> Switch1/3
  Divide1/1 -> Integrator8/1  "yl''"
  Fhw1/1 -> Gain16/1
  Product8/1 -> Sum16/2
  Sin/1 -> Product7/1
  Sum16/1 -> Sum18/1

== system PlantaV4_6_prueba_contacto_4/whd*(t)1 ==
  Demux : Demux  Tag=STV Demux  Outputs=1
      settings: DisplayOption=none
  FromWs : FromWorkspace  Tag=STV FromWs  VariableName=tuvar
      SigBuilderData=|
      | common.afterFinalStr = 'Extrapolate'
      | common.sampleTime = 0
      | dataSet.timeRange = [0 100]
      | dataSet.name = 'Group 1'
      | sbobj.Groups.Name = 'Group 1'
      | sbobj.Groups.Signals.Name = 'Signal 2'
      | sbobj.Groups.Signals.XData = [0 10 20 25 60 100]
      | sbobj.Groups.Signals.YData = [0 1 1 0 0 0]
      | sbobj.Groups.TimeRange = [0 100]
  Signal 2 : Outport  Tag=STV Outport
  wires:
  FromWs/1 -> Demux/1
  Demux/1 -> Signal 2/1

== system PlantaV4_6_prueba_contacto_4/whd*(t)2 ==
  Demux : Demux  Tag=STV Demux  Outputs=1
      settings: DisplayOption=none
  FromWs : FromWorkspace  Tag=STV FromWs  VariableName=tuvar
      SigBuilderData=|
      | common.afterFinalStr = 'Extrapolate'
      | common.sampleTime = 0
      | dataSet.timeRange = [0 100]
      | dataSet.name = 'Group 1'
      | sbobj.Groups.Name = 'Group 1'
      | sbobj.Groups.Signals.Name = 'Signal 2'
      | sbobj.Groups.Signals.XData = [0 10 20 25 60 100]
      | sbobj.Groups.Signals.YData = [0 1 1 0 0 0]
      | sbobj.Groups.TimeRange = [0 100]
  Signal 2 : Outport  Tag=STV Outport
  wires:
  FromWs/1 -> Demux/1
  Demux/1 -> Signal 2/1

== stateflow chart PlantaV4_6_prueba_contacto_4/Frenos Traslación ==
  state FrenosOperacion
    state BRKt_off
      during:
      Ttb=-btb*wtm;
      Ttb=min(Ttb_Max,max(-Ttb_Max, Ttb));
    state BRKt_on
      during:
      Ttb=0;
    (default) -> BRKt_off
    BRKt_off -> BRKt_on : [BRKt==1 ]
    BRKt_on -> BRKt_off : [BRKt==0]
  data: Ttb output; wtm input; btb parameter; BRKt input; Ttb_Max input

== stateflow chart PlantaV4_6_prueba_contacto_4/Chart ==
  state Masa
    entry:
    Mcx = fcn(Mc_max, Mc_min);
  data: Mc_MAX function_input; Mc_MIN function_input; ML function_output; Mc_max parameter; Mcx output; Mc_min parameter; flag_carga local
  function ML = fcn(Mc_MAX, Mc_MIN):
    | function ML = fcn(Mc_MAX, Mc_MIN)
    | %Agregar: sobrecarga
    | %if (flag_carga == 1)
    |     ML = Mc_MIN + (Mc_MAX - Mc_MIN)*rand(1);
    |     %ml = Mc_Max + 0.01 * randi([1,15],1) * Mc_Max;
    | %else
    |  %   ML = 0;
    | %end
    | end

== stateflow chart PlantaV4_6_prueba_contacto_4/Frenos Izaje  ==
  state FrenosOperacion
    state BRKh_off
      during:
      Thb=-bhb*whm;
      Thb=min(Thb_Max,max(-Thb_Max,Thb ));
    state BRKh_on
      during:
      Thb=0;
    (default) -> BRKh_off
    BRKh_off -> BRKh_on [order 1] : [BRKh==1 && BRKhE==1]
    BRKh_on -> BRKh_off [order 1] : [BRKh==0 && BRKhE==1]
  state FrenosEmergencia
    state BRKhE_off
      during:
      ThEb=-bhEb*whd;
      ThEb=min(ThEb_Max,max(-ThEb_Max, ThEb));
    state BRKhE_on
      during:
      ThEb=0;
    (default) -> BRKhE_off
    BRKhE_off -> BRKhE_on : [BRKhE==1]
    BRKhE_on -> BRKhE_off [order 1] : [BRKhE==0]
  BRKh_on -> FrenosEmergencia [order 2] : [BRKhE==0]
  BRKh_off -> FrenosEmergencia [order 2] : [BRKhE==0]
  BRKhE_on -> FrenosOperacion [order 2] : [BRKhE==1]
  (default) -> FrenosEmergencia
  data: whm input; bhb parameter; BRKh input; bhEb parameter; BRKhE input; Thb output; ThEb output; Thb_Max parameter; ThEb_Max parameter; whd input

== stateflow chart PlantaV4_6_prueba_contacto_4/Chart1 ==
  state Balanceo
    during:
    [KP,KD,WN]=balanceo(Meq, Mt,ml,l,g)
    %[KP,KD,KI,WN]=balanceo(ml, Mt, g, l)
  (default) -> Balanceo
  data: MEQ function_input; mt function_input; Ml function_input; L function_input; G function_input; Kd function_output; Kp function_output; wn function_output; l input; ml input; KD output; KP output; g parameter; Meq parameter; WN output; Mt parameter
  function [Kd,Kp, wn]=balanceo(MEQ, mt,Ml,L,G):
    | function [Kd,Kp, wn]=balanceo(MEQ, mt,Ml,L,G)
    |     
    | %     Kd=(1+(L*(mt+Ml)))/(mt+Ml);
    | %     Kp=(2*0.7*wn)/(mt+Ml);
    | %     w=((mt*G/((mt+Ml)*L))^0.5);
    | %     Kd=(mt*G/w^2 + (mt+Ml)*L)/(Ml+mt);
    | %     Kp=2*0.7*(-(mt+Ml)*L/(Ml+mt)+Kd);
    |     
    |     %correccion agustin
    |     %wn=((mt*G)/(L*(mt+Ml)))^(0.5);
    |     %Kd = L - (mt*G)/((mt+Ml)*wn^2);
    |     %Kp = (2*z*wn)/(L-Kd);
    |     %correcion matias
    |     z = 0.9;
    |     wn=((MEQ*G)/(L*(MEQ+Ml)))^(0.5);
    |     wn = 1 * wn; %el mejor: 2
    |     Kd = ((-MEQ*G)/(wn^2) +(MEQ+Ml)*L)* 1/(mt+Ml);
    |     Kp = (2*z*wn)*((MEQ+Ml)* L - Kd*(mt+Ml))/(mt+Ml);
    | end
    |  
    | % function [kp,kd,ki,wn] = balanceo(Ml,mt,G,L)
    | %     xita=0.9;%0.7;
    | %     wn=(mt*G/((mt+Ml)*L))^(1/2);
    | %     kd=-(mt*G/((mt+Ml)*(wn^(3))));
    | %     kp=(kd*(2*xita*wn-wn)+l);
    | %     ki=wn^2*(1-xita)*kd;
    | % end

== stateflow chart PlantaV4_6_prueba_contacto_4/Chart2 ==
  state Balanceo
    during:
    [KP,KD,KI,WN]=balanceoPID(Meq, Mt,ml,l,g)
    %[KP,KD,KI,WN]=balanceo(ml, Mt, g, l)
  (default) -> Balanceo
  data: MEQ function_input; mt function_input; Ml function_input; L function_input; G function_input; Kd function_output; Kp function_output; Ki function_output; wn function_output; l input; ml input; KD output; KP output; g parameter; Meq parameter; WN output; Mt parameter; KI output
  function [Kd,Kp,Ki,wn]=balanceoPID(MEQ, mt,Ml,L,G):
    | function [Kd,Kp,Ki,wn]=balanceoPID(MEQ, mt,Ml,L,G)
    |     
    | %     Kd=(1+(L*(mt+Ml)))/(mt+Ml);
    | %     Kp=(2*0.7*wn)/(mt+Ml);
    | %     w=((mt*G/((mt+Ml)*L))^0.5);
    | %     Kd=(mt*G/w^2 + (mt+Ml)*L)/(Ml+mt);
    | %     Kp=2*0.7*(-(mt+Ml)*L/(Ml+mt)+Kd);
    |     
    |     %correccion agustin
    |     %wn=((mt*G)/(L*(mt+Ml)))^(0.5);
    |     %Kd = L - (mt*G)/((mt+Ml)*wn^2);
    |     %Kp = (2*z*wn)/(L-Kd);
    |     %correcion matias
    |     z = 0.7;
    |     wn=((MEQ*G)/(L*(MEQ+Ml)))^(0.5);
    |     wn = 1 * wn; %el mejor: 2
    |     Ki = ((wn^2)*(Meq*L + Ml*(L+Kd)- Kd*mt) - MEQ*G)/(Ml-mt);
    |     Kp = ((2*z*wn)*((MEQ* L) - Ml*(L+Kd)-(Kd*mt)))/(Ml-mt);
    |     Kd = ((-MEQ*G)/(wn^2) +(MEQ+Ml)*L)* 1/(mt+Ml);    %cambiar
    | end
    |  
    | % function [kp,kd,ki,wn] = balanceo(Ml,mt,G,L)
    | %     xita=0.9;%0.7;
    | %     wn=(mt*G/((mt+Ml)*L))^(1/2);
    | %     kd=-(mt*G/((mt+Ml)*(wn^(3))));
    | %     kp=(kd*(2*xita*wn-wn)+l);
    | %     ki=wn^2*(1-xita)*kd;
    | % end

== stateflow chart PlantaV4_6_prueba_contacto_4/Chart3 ==
  state Balanceo
    during:
    [KI,KP,WN]=balanceoPI(Meq, Mt,ml,l,g)
    %[KP,KD,KI,WN]=balanceo(ml, Mt, g, l)
  (default) -> Balanceo
  data: MEQ function_input; mt function_input; Ml function_input; L function_input; G function_input; Ki function_output; Kp function_output; wn function_output; l input; ml input; KP output; g parameter; Meq parameter; WN output; Mt parameter; KI output
  function [Ki,Kp, wn]=balanceoPI(MEQ, mt,Ml,L,G):
    | function [Ki,Kp,wn]=balanceoPI(MEQ, mt,Ml,L,G)
    | 
    |     z = 0.9;
    |     wn=((MEQ*G)/(L*(MEQ+Ml)))^(0.5);
    |     wn = 1 * wn; %el mejor: 2
    |     Ki = ((wn^2)* ((MEQ+Ml)*L)- MEQ*G)/(mt+Ml);
    |     Kp = (2*z*wn)*((MEQ+Ml)* L )/(mt+Ml);
    | end

== stateflow chart PlantaV4_6_prueba_contacto_4/Enclavamiento carro ==
  (default) -> (junction 9) : % activacion de frenos
  (junction 9) -> (junction 4) [order 1] : [abs(wtm)<wtmMax]
  (junction 9) -> (junction 10) [order 2] : {BRKt=0;}
  (junction 4) -> (junction 2) : {BRKt=1;}
  (junction 2) -> (junction 10)
  (junction 10) -> (junction 11)
  data: wtmMax parameter; wtm input; BRKt output

== stateflow chart PlantaV4_6_prueba_contacto_4/Enclavamiento izaje ==
  (default) -> (junction 9) : % activacion de frenos
  (junction 9) -> (junction 4) [order 1] : [abs(whm)<whmMax]
  (junction 9) -> (junction 10) [order 2] : {BRKh=0;}
  (junction 4) -> (junction 2) : {BRKh=1;}
  (junction 2) -> (junction 10)
  (junction 10) -> (junction 11)
  data: whm input; BRKh output; whmMax parameter

== matlab function PlantaV4_6_prueba_contacto_4/MATLAB Function ==
  data: index output; estado_cont input; y_evol output; xl input; anchoCont input
function [index, y_evol] = envolvente(estado_cont, xl, anchoCont)
%Calculo de envolvente. Hay un perfil de contenedores. 
%Se debe usar la posicion actual de la carga para comparar con la altura
%que debe tener el contenedor (teniendo en cuenta el indice del vector)
%si la carga esta entre los limites del contenedor(i) (contenedor(i) -
%contenedor(i)aX*0.5 y contenedor(i) + contenedor(i)aX*0.5)
% Dividir la posicion en x de la carga por el ancho de contenedores para
% obtener la posicion del indice  (usar floor?) --> si da 0 por ejemplo la
% la altura del envolvente sera igual a la del contenedor en el indice 0
% mas el factor de seguridad. Para el modo de contacto no usar el factor de
% seguridad.
fseg = 0;  %2.5;  Buscar si no esta guardado previamente
index = floor((xl)/anchoCont)+1;   %revisar +1
%si xl es menor a 0 (con las posiciones corregidas, sin el offset,
%modificar los valores para que sean 0 (muelle) o la altura de un camion

%% index: puedo hacer que compare index con index anterior
    if (index<=0)
        y_evol = 0; %-6+fseg; %por ahora solo muelle, si uso 0 entra directo en modo contancto

    elseif (index>0 && index<=20)
    %     y_evol = con(index) + fseg;
        y_evol = estado_cont(2,index) + fseg;
    elseif (index>20)
        %no deberia pasar 
        y_evol = -5+fseg;
    else
        y_evol = 0;
    end


end

== stateflow chart PlantaV4_6_prueba_contacto_4/graficos ==
  state Graficar
    entry:
    cont = 0;
    %contenedor = rectangle('Position',[xl-2.25, yl, 4.5, 2.5 ],'FaceColor','g');
    %carro = rectangle('Position',[xt-2, Yt0, 4.5, 2 ],'FaceColor','r');
    during:
    dock_shore_graph(xt, xl, yl, Yt0,Hc,cont);
    cont = cont+1;
  (default) -> Graficar
  data: Xt function_input; Xl function_input; Yl function_input; YT0 function_input; HC function_input; Con function_input; Hc input; Yt0 input; xl input; xt input; yl input; cont local
  function dock_shore_graph(Xt, Xl, Yl, YT0, HC,Con):
    | function dock_shore_graph(Xt, Xl, Yl, YT0, HC,Con)
    | %viga voladiza
    | plot([-30 50],[45 45 ],'Color','k')
    | hold on
    | %cable
    | cable = plot([xt xl],[45 yl+Hc],'Color','k');
    | %carro (modificar luego)
    | carro = rectangle('Position',[xt-2, Yt0, 4.5, 2 ],'FaceColor','r');
    | %Conenedor
    | contenedor = rectangle('Position',[xl-2.25, yl, 4.5, 2.5 ],'FaceColor','g');
    | %barco
    | rectangle('Position',[2, -20.5, 0.5, 25.5 ],'FaceColor','b');
    | rectangle('Position',[50, -20.5, 0.5, 25.5 ],'FaceColor','b');
    | rectangle('Position',[2, -20.5, 48, 0.5 ],'FaceColor','b');
    | %muelle
    | rectangle('Position',[-30, -0.5, 30, 0.5 ],'FaceColor','k');
    | rectangle('Position',[0, -20, 0.5, 20 ],'FaceColor','k');
    | 
    | title("Operacion de carga y descarga");
    | xlabel("Distancia (mts)");
    | ylabel("Altura (mts)");
    | hold on
    | if (cont>0)
    |     set(carro, 'Position', [xt-2, Yt0, 4.5, 2 ]);
    |     set(contenedor, 'Position', [xl-2.25, yl, 4.5, 2.5 ]);
    |     set(cable,'XData', [xt xl], 'YData', [45 yl]);
    |     %cable = plot([xt xl],[45 yl],'Color','k');
    | end
    | % %perfil de contenedores VARIABLE
    | % x = 6.5:5:46.5;
    | % y = [15 20 32 16 35 11 32 22 10];
    | % b = bar(x,y); %,'histc'
    | % b(1).BaseValue = -20;
    | % b(1).BaseLine.LineWidth = 0.01;
    | % b(1).ShowBaseLine=0;
    | % b(1).BarWidth=0.9;
    | % b(1).FaceColor = [0.8500 0.3250 0.0980];
    | % % Actualizar los datos del gráfico de barras
    | % set(b, 'YData', datos);
    | %---------------------------------------------------
    | % Perfil de contenedores
    | puntos_iniciales = [5 -20; 10 -20; 15 -20; 20 -20; 25 -20; 30 -20; 35 -20; 40 -20; 45 -20];
    | % Definir las dimensiones de los rectángulos
    | dimensiones = [15; 12; 20; 18; 14; 16; 13; 10; 8];
    | 
    | % Bucle para crear los rectángulos
    | for i = 1:size(puntos_iniciales, 1)
    |     % Obtener las coordenadas del punto inicial
    |     x = puntos_iniciales(i, 1);
    |     y = puntos_iniciales(i, 2);
    |     altura = dimensiones(i);
    |     % Crear el rectángulo utilizando el comando 'rectangle'
    |     rectangle('Position', [x, y, 5, altura], 'FaceColor', 'red');
    |     
    | %     hold on; % Para mantener los rectángulos en el gráfico
    | end
    | 
    | % Refrescar el gráfico
    | drawnow;
    | 
    | % Pausa para observar el cambio en el gráfico
    | pause(0.5);
    | set(carro, 'visible', 'off');
    | set(contenedor, 'visible', 'off');
    | set(cable, 'visible', 'off');
    | % if (mod(cont,7)==0)
    | %     set(carro, 'visible', 'off');
    | %     set(contenedor, 'visible', 'off');
    | %     %carro (modificar luego)
    | % carro = rectangle('Position',[xt-2, Yt0, 4.5, 2 ],'FaceColor','r');
    | % %Conenedor
    | % contenedor = rectangle('Position',[xl-2.25, yl, 4.5, 2.5 ],'FaceColor','g');
    | % end
    | end

== stateflow chart PlantaV4_6_prueba_contacto_4/Modo Twistlocks ==
  state TLK_OFF
    entry:
    hc=0;
    ml=Ms;
  state TLK_ON
    entry:
    hc=2.5;
    ml=Ms+Mcx;
  (default) -> TLK_OFF
  TLK_OFF -> TLK_ON : [Mcx>0]
  TLK_ON -> TLK_OFF : [Mcx<=0]
  data: Mcx input; hc output; ml output; Ms parameter
